simulink model "Problem4"  (R2020b)
settings: Solver=VariableStepAuto  StartTime=0.0  StopTime=10.0  RelTol=1e-3
settings Model: Creator=Akshata Ashok  LastModifiedBy=Akshata Ashok

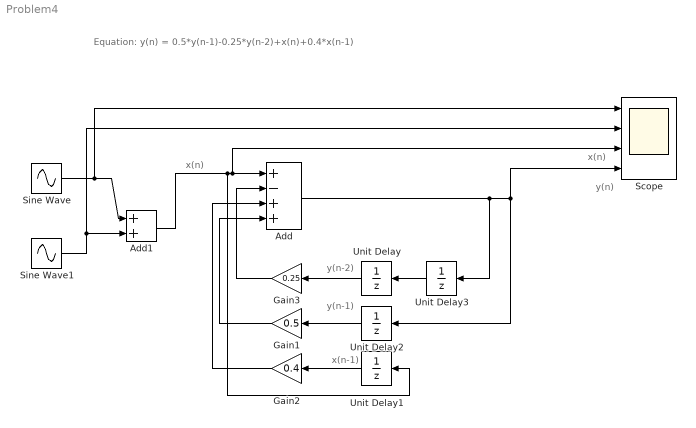
== system Problem4 ==
  note: y(n)
  note: x(n)
  note: Equation:
      | y(n) = 0.5*y(n-1)-0.25*y(n-2)+x(n)+0.4*x(n-1)
  note: y(n-2)
  note: y(n-1)
  note: x(n-1)
  note: x(n)
  Add : Sum  Inputs=+-++
  Add1 : Sum
  Gain1 : Gain  Gain=0.5
  Gain2 : Gain  Gain=0.4
  Gain3 : Gain  Gain=0.25
  Scope : Scope  NumInputPorts=4
  Sine Wave : Sin  Amplitude=0.5  Frequency=50  SampleTime=0
  Sine Wave1 : Sin  SampleTime=0
  Unit Delay{,1..3} (4 alike) : UnitDelay  SampleTime=-1  HasFrameUpgradeWarning=on
  wires:
  Unit Delay/1 -> Gain3/1
  Unit Delay2/1 -> Gain1/1
  Unit Delay3/1 -> Unit Delay/1
  Add/1 -> Unit Delay3/1, Unit Delay2/1, Scope/4
  Gain2/1 -> Add/3
  Unit Delay1/1 -> Gain2/1
  Gain1/1 -> Add/4
  Gain3/1 -> Add/2
  Sine Wave/1 -> Scope/1, Add1/1
  Sine Wave1/1 -> Scope/2, Add1/2
  Add1/1 -> Add/1, Scope/3, Unit Delay1/1
